simulink model "chap05"  (R2021a)
settings: Solver=FixedStepDiscrete  StartTime=0.0  StopTime=inf  FixedStep=0.001  RelTol=1e-3
undefined symbols (not defined in the file): DiscIntNeverNeededParam, Header, Pose, X, Y, Z
libraries: robotlib x31
(part 5 of 9)

== system chap05/Subsystem16/Subsystem12/Subsystem1 ==
  xx6 : Inport
  xx0 : Inport  Port=2
  xx1 : Inport  Port=3
  xx2 : Inport  Port=4
  vx6 : Inport  Port=5
  vx0 : Inport  Port=6
  vx1 : Inport  Port=7
  vx2 : Inport  Port=8
  Add : Sum
  Add1 : Sum  Inputs=-+
  Add10 : Sum  Inputs=-+
  Add2 : Sum  Inputs=+-
  Add4 : Sum  Inputs=-+
  Add5 : Sum  Inputs=+++
  Add6 : Sum  Inputs=+-
  Add8 : Sum  Inputs=+++
  Add9 : Sum  Inputs=+-
  Constant : Constant  Value=0.75
  Constant1 : Constant  Value=0.85
  Constant3 : Constant  Value=1.2
  Constant{4..5,7..8} (4 alike) : Constant  Value=1.5
  Constant6 : Constant  Value=1.2
  Product{1,3..9} (8 alike) : Product
  utx : Outport
  wires:
  Product7/1 -> Add8/3
  Add6/1 -> Product7/1
  Constant8/1 -> Product7/2
  vx0/1 -> Add6/2
  Product3/1 -> Add5/1
  Add1/1 -> Product3/2
  Constant7/1 -> Product3/1
  xx0/1 -> Add1/1
  vx6/1 -> Add10/2, Add9/1, Add6/1
  vx2/1 -> Add10/1
  vx1/1 -> Add9/2
  xx1/1 -> Add2/2
  xx2/1 -> Add4/1
  Add/1 -> utx/1
  Add5/1 -> Product6/2
  Add2/1 -> Product5/1
  Product1/1 -> Add/2
  Constant1/1 -> Product1/1
  Constant/1 -> Product6/1
  Product6/1 -> Add/1
  Constant3/1 -> Product5/2
  xx6/1 -> Add4/2, Add2/1, Add1/2
  Add4/1 -> Product4/2
  Constant4/1 -> Product4/1
  Product5/1 -> Add5/3
  Product4/1 -> Add5/2
  Add8/1 -> Product1/2
  Constant5/1 -> Product8/1
  Add10/1 -> Product8/2
  Constant6/1 -> Product9/2
  Add9/1 -> Product9/1
  Product8/1 -> Add8/1
  Product9/1 -> Add8/2

== system chap05/Subsystem16/Subsystem12/Subsystem2 ==
  xx6 : Inport
  xx0 : Inport  Port=2
  xx1 : Inport  Port=3
  xx2 : Inport  Port=4
  vx6 : Inport  Port=5
  vx0 : Inport  Port=6
  vx1 : Inport  Port=7
  vx2 : Inport  Port=8
  Add : Sum
  Add1 : Sum  Inputs=-+
  Add10 : Sum  Inputs=-+
  Add2 : Sum  Inputs=+-
  Add4 : Sum  Inputs=-+
  Add5 : Sum  Inputs=+++
  Add6 : Sum  Inputs=+-
  Add8 : Sum  Inputs=+++
  Add9 : Sum  Inputs=+-
  Constant : Constant  Value=0.75
  Constant1 : Constant  Value=0.85
  Constant3 : Constant  Value=1.2
  Constant{4..5,7..8} (4 alike) : Constant  Value=1.5
  Constant6 : Constant  Value=1.2
  Product{1,3..9} (8 alike) : Product
  utx : Outport
  wires:
  Product9/1 -> Add8/2
  Product8/1 -> Add8/1
  Add9/1 -> Product9/1
  Constant6/1 -> Product9/2
  Add10/1 -> Product8/2
  Constant5/1 -> Product8/1
  Add8/1 -> Product1/2
  Product4/1 -> Add5/2
  Product5/1 -> Add5/3
  Constant4/1 -> Product4/1
  Add4/1 -> Product4/2
  xx6/1 -> Add1/2, Add2/1, Add4/2
  Constant3/1 -> Product5/2
  Product6/1 -> Add/1
  Constant/1 -> Product6/1
  Constant1/1 -> Product1/1
  Product1/1 -> Add/2
  Add2/1 -> Product5/1
  Add5/1 -> Product6/2
  Add/1 -> utx/1
  xx2/1 -> Add4/1
  xx1/1 -> Add2/2
  vx1/1 -> Add9/2
  vx2/1 -> Add10/1
  vx6/1 -> Add6/1, Add9/1, Add10/2
  xx0/1 -> Add1/1
  Constant7/1 -> Product3/1
  Add1/1 -> Product3/2
  Product3/1 -> Add5/1
  vx0/1 -> Add6/2
  Constant8/1 -> Product7/2
  Add6/1 -> Product7/1
  Product7/1 -> Add8/3

== system chap05/Subsystem16/Subsystem12/Subsystem3 ==
  xyk : Inport
  xy : Inport  Port=2
  vyk : Inport  Port=3
  vy : Inport  Port=4
  Add : Sum
  Add4 : Sum  Inputs=-+
  Add8 : Sum  Inputs=-+
  Constant : Constant  Value=0.75
  Constant1 : Constant  Value=0.85
  Product1 : Product
  Product6 : Product
  ey : Outport
  wires:
  vyk/1 -> Add8/2
  vy/1 -> Add8/1
  xy/1 -> Add4/1
  Add/1 -> ey/1
  Add4/1 -> Product6/2
  Product1/1 -> Add/2
  Constant1/1 -> Product1/1
  Constant/1 -> Product6/1
  Product6/1 -> Add/1
  xyk/1 -> Add4/2
  Add8/1 -> Product1/2

== system chap05/Subsystem16/Subsystem12/Subsystem4 ==
  xzk : Inport
  xz : Inport  Port=2
  vzk : Inport  Port=3
  vz : Inport  Port=4
  Add : Sum
  Add4 : Sum  Inputs=-+
  Add8 : Sum  Inputs=-+
  Constant : Constant  Value=0.75
  Constant1 : Constant  Value=0.85
  Product1 : Product
  Product6 : Product
  ez : Outport
  wires:
  Add8/1 -> Product1/2
  xzk/1 -> Add4/2
  Product6/1 -> Add/1
  Constant/1 -> Product6/1
  Constant1/1 -> Product1/1
  Product1/1 -> Add/2
  Add4/1 -> Product6/2
  Add/1 -> ez/1
  xz/1 -> Add4/1
  vz/1 -> Add8/1
  vzk/1 -> Add8/2

== system chap05/Subsystem16/Subsystem12/Subsystem5 ==
  xxk : Inport
  xx : Inport  Port=2
  vxk : Inport  Port=3
  vx : Inport  Port=4
  Add : Sum
  Add4 : Sum  Inputs=-+
  Add8 : Sum  Inputs=-+
  Constant : Constant  Value=0.75
  Constant1 : Constant  Value=0.85
  Product1 : Product
  Product6 : Product
  ex : Outport
  wires:
  Add8/1 -> Product1/2
  xxk/1 -> Add4/2
  Product6/1 -> Add/1
  Constant/1 -> Product6/1
  Constant1/1 -> Product1/1
  Product1/1 -> Add/2
  Add4/1 -> Product6/2
  Add/1 -> ex/1
  xx/1 -> Add4/1
  vx/1 -> Add8/1
  vxk/1 -> Add8/2

== system chap05/Subsystem16/Subsystem12/Subsystem6 ==
  xx6 : Inport
  xx0 : Inport  Port=2
  xx1 : Inport  Port=3
  xx2 : Inport  Port=4
  vx6 : Inport  Port=5
  vx0 : Inport  Port=6
  vx1 : Inport  Port=7
  vx2 : Inport  Port=8
  Add : Sum
  Add1 : Sum  Inputs=-+
  Add10 : Sum  Inputs=-+
  Add2 : Sum  Inputs=+-
  Add4 : Sum  Inputs=-+
  Add5 : Sum  Inputs=+++
  Add6 : Sum  Inputs=+-
  Add8 : Sum  Inputs=+++
  Add9 : Sum  Inputs=+-
  Constant : Constant  Value=0.75
  Constant1 : Constant  Value=0.85
  Constant3 : Constant  Value=1.2
  Constant{4..5,7..8} (4 alike) : Constant  Value=1.5
  Constant6 : Constant  Value=1.2
  Product{1,3..9} (8 alike) : Product
  utx : Outport
  wires:
  Product9/1 -> Add8/2
  Product8/1 -> Add8/1
  Add9/1 -> Product9/1
  Constant6/1 -> Product9/2
  Add10/1 -> Product8/2
  Constant5/1 -> Product8/1
  Add8/1 -> Product1/2
  Product4/1 -> Add5/2
  Product5/1 -> Add5/3
  Constant4/1 -> Product4/1
  Add4/1 -> Product4/2
  xx6/1 -> Add1/2, Add2/1, Add4/2
  Constant3/1 -> Product5/2
  Product6/1 -> Add/1
  Constant/1 -> Product6/1
  Constant1/1 -> Product1/1
  Product1/1 -> Add/2
  Add2/1 -> Product5/1
  Add5/1 -> Product6/2
  Add/1 -> utx/1
  xx2/1 -> Add4/1
  xx1/1 -> Add2/2
  vx1/1 -> Add9/2
  vx2/1 -> Add10/1
  vx6/1 -> Add6/1, Add9/1, Add10/2
  xx0/1 -> Add1/1
  Constant7/1 -> Product3/1
  Add1/1 -> Product3/2
  Product3/1 -> Add5/1
  vx0/1 -> Add6/2
  Constant8/1 -> Product7/2
  Add6/1 -> Product7/1
  Product7/1 -> Add8/3

== system chap05/Subsystem16/Subsystem14/L+B ==
  Add : Sum
  Constant1 : Constant  Value=|
      | [2.5 0 0 0 0 0
      |      0 2.8 0 0 0 0
      |      0 0 2.8 0 0 0
      |      0 0 0 2.5 0 0
      |      0 0 0 0 2.7 0
      |      0 0 0 0 0 2.7]
  Constant2 : Constant  Value=|
      | [0.0 0.8 0.5 0.0 0.0 1.2
      |      0.8 0.0 0.0 0.5 0.0 1.5
      |      0.5 0.0 0.0 0.8 1.5 0.0
      |      0.0 0.5 0.8 0.0 1.2 0.0
      |      0.0 0.0 1.5 1.2 0.0 0.0
      |      1.2 1.5 0.0 0.0 0.0 0.0]
  Constant3 : Constant  Value=|
      | [0.0 0.0 0.0 0.0 0.0 0.0
      |      0.0 0.0 0.0 0.0 0.0 0.0
      |      0.0 0.0 0.0 0.0 0.0 0.0
      |      0.0 0.0 0.0 0.0 0.0 0.0
      |      0.0 0.0 0.0 0.0 1.5 0.0
      |      0.0 0.0 0.0 0.0 0.0 1.5]
  Subtract : Sum  Inputs=+-
  u : Outport
  wires:
  Constant2/1 -> Subtract/2
  Constant1/1 -> Subtract/1
  Subtract/1 -> Add/1
  Add/1 -> u/1
  Constant3/1 -> Add/2

== system chap05/Subsystem16/Subsystem14/Subsystem1 ==
  xy1 : Inport
  xy2 : Inport  Port=2
  xy3 : Inport  Port=3
  xy6 : Inport  Port=4
  vy1 : Inport  Port=5
  vy2 : Inport  Port=6
  vy3 : Inport  Port=7
  vy6 : Inport  Port=8
  Add : Sum
  Add{1,4,6,8} (4 alike) : Sum  Inputs=-+
  Add2 : Sum  Inputs=+-
  Add5 : Sum  Inputs=+++
  Add7 : Sum  Inputs=+-
  Add9 : Sum  Inputs=+++
  Constant : Constant  Value=0.75
  Constant1 : Constant  Value=0.85
  Constant3 : Constant  Value=0.5
  Constant4 : Constant  Value=0.8
  Constant5 : Constant  Value=1.2
  Constant7 : Constant  Value=0.5
  Constant8 : Constant  Value=0.8
  Constant9 : Constant  Value=1.2
  Product{1,3..9} (8 alike) : Product
  p2y : Outport
  wires:
  Add9/1 -> Product1/2
  Product4/1 -> Add5/2
  Product5/1 -> Add5/3
  Constant3/1 -> Product4/1
  Add4/1 -> Product4/2
  xy1/1 -> Add1/2, Add4/2, Add2/1
  Constant4/1 -> Product5/2
  Product6/1 -> Add/1
  Constant/1 -> Product6/1
  Constant1/1 -> Product1/1
  Product1/1 -> Add/2
  Add2/1 -> Product5/1
  Add5/1 -> Product6/2
  Add/1 -> p2y/1
  xy3/1 -> Add4/1
  xy2/1 -> Add2/2
  xy6/1 -> Add1/1
  Constant5/1 -> Product3/1
  Add1/1 -> Product3/2
  Product3/1 -> Add5/1
  Product7/1 -> Add9/1
  Add6/1 -> Product7/2
  Constant9/1 -> Product7/1
  vy6/1 -> Add6/1
  vy2/1 -> Add7/2
  vy3/1 -> Add8/1
  Add7/1 -> Product9/1
  Constant8/1 -> Product9/2
  vy1/1 -> Add7/1, Add8/2, Add6/2
  Add8/1 -> Product8/2
  Constant7/1 -> Product8/1
  Product9/1 -> Add9/3
  Product8/1 -> Add9/2

== system chap05/Subsystem16/Subsystem14/Subsystem2 ==
  xz1 : Inport
  xx2 : Inport  Port=2
  xz3 : Inport  Port=3
  xz6 : Inport  Port=4
  vz1 : Inport  Port=5
  vz2 : Inport  Port=6
  vz3 : Inport  Port=7
  vz6 : Inport  Port=8
  Add : Sum
  Add{1,4,6,8} (4 alike) : Sum  Inputs=-+
  Add2 : Sum  Inputs=+-
  Add5 : Sum  Inputs=+++
  Add7 : Sum  Inputs=+-
  Add9 : Sum  Inputs=+++
  Constant : Constant  Value=0.75
  Constant1 : Constant  Value=0.85
  Constant3 : Constant  Value=0.5
  Constant4 : Constant  Value=0.8
  Constant5 : Constant  Value=1.2
  Constant7 : Constant  Value=0.5
  Constant8 : Constant  Value=0.8
  Constant9 : Constant  Value=1.2
  Product{1,3..9} (8 alike) : Product
  p3z : Outport
  wires:
  Product8/1 -> Add9/2
  Product9/1 -> Add9/3
  Constant7/1 -> Product8/1
  Add8/1 -> Product8/2
  vz1/1 -> Add6/2, Add8/2, Add7/1
  Constant8/1 -> Product9/2
  Add7/1 -> Product9/1
  vz3/1 -> Add8/1
  vz2/1 -> Add7/2
  vz6/1 -> Add6/1
  Constant9/1 -> Product7/1
  Add6/1 -> Product7/2
  Product7/1 -> Add9/1
  Product3/1 -> Add5/1
  Add1/1 -> Product3/2
  Constant5/1 -> Product3/1
  xz6/1 -> Add1/1
  xx2/1 -> Add2/2
  xz3/1 -> Add4/1
  Add/1 -> p3z/1
  Add5/1 -> Product6/2
  Add2/1 -> Product5/1
  Product1/1 -> Add/2
  Constant1/1 -> Product1/1
  Constant/1 -> Product6/1
  Product6/1 -> Add/1
  Constant4/1 -> Product5/2
  xz1/1 -> Add2/1, Add4/2, Add1/2
  Add4/1 -> Product4/2
  Constant3/1 -> Product4/1
  Product5/1 -> Add5/3
  Product4/1 -> Add5/2
  Add9/1 -> Product1/2

== system chap05/Subsystem16/Subsystem14/Subsystem3 ==
  xyk : Inport
  xy : Inport  Port=2
  vyk : Inport  Port=3
  vy : Inport  Port=4
  Add : Sum
  Add4 : Sum  Inputs=-+
  Add8 : Sum  Inputs=-+
  Constant : Constant  Value=0.75
  Constant1 : Constant  Value=0.85
  Product1 : Product
  Product6 : Product
  ey : Outport
  wires:
  vyk/1 -> Add8/2
  vy/1 -> Add8/1
  xy/1 -> Add4/1
  Add/1 -> ey/1
  Add4/1 -> Product6/2
  Product1/1 -> Add/2
  Constant1/1 -> Product1/1
  Constant/1 -> Product6/1
  Product6/1 -> Add/1
  xyk/1 -> Add4/2
  Add8/1 -> Product1/2

== system chap05/Subsystem16/Subsystem14/Subsystem4 ==
  xzk : Inport
  xz : Inport  Port=2
  vzk : Inport  Port=3
  vz : Inport  Port=4
  Add : Sum
  Add4 : Sum  Inputs=-+
  Add8 : Sum  Inputs=-+
  Constant : Constant  Value=0.75
  Constant1 : Constant  Value=0.85
  Product1 : Product
  Product6 : Product
  ez : Outport
  wires:
  Add8/1 -> Product1/2
  xzk/1 -> Add4/2
  Product6/1 -> Add/1
  Constant/1 -> Product6/1
  Constant1/1 -> Product1/1
  Product1/1 -> Add/2
  Add4/1 -> Product6/2
  Add/1 -> ez/1
  xz/1 -> Add4/1
  vz/1 -> Add8/1
  vzk/1 -> Add8/2

== system chap05/Subsystem16/Subsystem14/Subsystem5 ==
  xxk : Inport
  xx : Inport  Port=2
  vxk : Inport  Port=3
  vx : Inport  Port=4
  Add : Sum
  Add4 : Sum  Inputs=-+
  Add8 : Sum  Inputs=-+
  Constant : Constant  Value=0.75
  Constant1 : Constant  Value=0.85
  Product1 : Product
  Product6 : Product
  ex : Outport
  wires:
  Add8/1 -> Product1/2
  xxk/1 -> Add4/2
  Product6/1 -> Add/1
  Constant/1 -> Product6/1
  Constant1/1 -> Product1/1
  Product1/1 -> Add/2
  Add4/1 -> Product6/2
  Add/1 -> ex/1
  xx/1 -> Add4/1
  vx/1 -> Add8/1
  vxk/1 -> Add8/2

== system chap05/Subsystem16/Subsystem14/Subsystem6 ==
  xx1 : Inport
  xx2 : Inport  Port=2
  xx3 : Inport  Port=3
  xx6 : Inport  Port=4
  vx1 : Inport  Port=5
  vx2 : Inport  Port=6
  vx3 : Inport  Port=7
  vx6 : Inport  Port=8
  Add : Sum
  Add{1,4,6,8} (4 alike) : Sum  Inputs=-+
  Add2 : Sum  Inputs=+-
  Add5 : Sum  Inputs=+++
  Add7 : Sum  Inputs=+-
  Add9 : Sum  Inputs=+++
  Constant : Constant  Value=0.75
  Constant1 : Constant  Value=0.85
  Constant3 : Constant  Value=0.5
  Constant4 : Constant  Value=0.8
  Constant5 : Constant  Value=1.2
  Constant7 : Constant  Value=0.5
  Constant8 : Constant  Value=0.8
  Constant9 : Constant  Value=1.2
  Product{1,3..9} (8 alike) : Product
  p1x : Outport
  wires:
  Product8/1 -> Add9/2
  Product9/1 -> Add9/3
  Constant7/1 -> Product8/1
  Add8/1 -> Product8/2
  vx1/1 -> Add6/2, Add8/2, Add7/1
  Constant8/1 -> Product9/2
  Add7/1 -> Product9/1
  vx3/1 -> Add8/1
  vx2/1 -> Add7/2
  vx6/1 -> Add6/1
  Constant9/1 -> Product7/1
  Add6/1 -> Product7/2
  Product7/1 -> Add9/1
  Product3/1 -> Add5/1
  Add1/1 -> Product3/2
  Constant5/1 -> Product3/1
  xx6/1 -> Add1/1
  xx2/1 -> Add2/2
  xx3/1 -> Add4/1
  Add/1 -> p1x/1
  Add5/1 -> Product6/2
  Add2/1 -> Product5/1
  Product1/1 -> Add/2
  Constant1/1 -> Product1/1
  Constant/1 -> Product6/1
  Product6/1 -> Add/1
  Constant4/1 -> Product5/2
  xx1/1 -> Add2/1, Add4/2, Add1/2
  Add4/1 -> Product4/2
  Constant3/1 -> Product4/1
  Product5/1 -> Add5/3
  Product4/1 -> Add5/2
  Add9/1 -> Product1/2

== system chap05/Subsystem16/Subsystem15/L+B ==
  Add : Sum
  Constant1 : Constant  Value=|
      | [2.5 0 0 0 0 0
      |      0 2.8 0 0 0 0
      |      0 0 2.8 0 0 0
      |      0 0 0 2.5 0 0
      |      0 0 0 0 2.7 0
      |      0 0 0 0 0 2.7]
  Constant2 : Constant  Value=|
      | [0.0 0.8 0.5 0.0 0.0 1.2
      |      0.8 0.0 0.0 0.5 0.0 1.5
      |      0.5 0.0 0.0 0.8 1.5 0.0
      |      0.0 0.5 0.8 0.0 1.2 0.0
      |      0.0 0.0 1.5 1.2 0.0 0.0
      |      1.2 1.5 0.0 0.0 0.0 0.0]
  Constant3 : Constant  Value=|
      | [0.0 0.0 0.0 0.0 0.0 0.0
      |      0.0 0.0 0.0 0.0 0.0 0.0
      |      0.0 0.0 0.0 0.0 0.0 0.0
      |      0.0 0.0 0.0 0.0 0.0 0.0
      |      0.0 0.0 0.0 0.0 1.5 0.0
      |      0.0 0.0 0.0 0.0 0.0 1.5]
  Subtract : Sum  Inputs=+-
  u : Outport
  wires:
  Constant2/1 -> Subtract/2
  Constant1/1 -> Subtract/1
  Subtract/1 -> Add/1
  Add/1 -> u/1
  Constant3/1 -> Add/2

== system chap05/Subsystem16/Subsystem15/Subsystem1 ==
  xy2 : Inport
  xy1 : Inport  Port=2
  xy4 : Inport  Port=3
  xy6 : Inport  Port=4
  vy2 : Inport  Port=5
  vy1 : Inport  Port=6
  vy4 : Inport  Port=7
  vy6 : Inport  Port=8
  Add : Sum
  Add{1,4,6,8} (4 alike) : Sum  Inputs=-+
  Add2 : Sum  Inputs=+-
  Add5 : Sum  Inputs=+++
  Add7 : Sum  Inputs=+-
  Add9 : Sum  Inputs=+++
  Constant : Constant  Value=0.75
  Constant1 : Constant  Value=0.85
  Constant2 : Constant  Value=0.5
  Constant3 : Constant  Value=0.5
  Constant4 : Constant  Value=0.8
  Constant5 : Constant  Value=1.5
  Constant6 : Constant  Value=0.8
  Constant7 : Constant  Value=1.5
  Product{1,3..9} (8 alike) : Product
  p2y : Outport
  wires:
  Product8/1 -> Add9/2
  Product9/1 -> Add9/3
  Constant2/1 -> Product8/1
  Add8/1 -> Product8/2
  vy2/1 -> Add6/2, Add8/2, Add7/1
  Constant6/1 -> Product9/2
  Add7/1 -> Product9/1
  vy4/1 -> Add8/1
  vy1/1 -> Add7/2
  vy6/1 -> Add6/1
  Constant7/1 -> Product7/1
  Add6/1 -> Product7/2
  Product7/1 -> Add9/1
  Product3/1 -> Add5/1
  Add1/1 -> Product3/2
  Constant5/1 -> Product3/1
  xy6/1 -> Add1/1
  xy1/1 -> Add2/2
  xy4/1 -> Add4/1
  Add5/1 -> Product6/2
  Add2/1 -> Product5/1
  Product1/1 -> Add/2
  Constant1/1 -> Product1/1
  Constant/1 -> Product6/1
  Product6/1 -> Add/1
  Constant4/1 -> Product5/2
  xy2/1 -> Add2/1, Add4/2, Add1/2
  Add4/1 -> Product4/2
  Constant3/1 -> Product4/1
  Product5/1 -> Add5/3
  Product4/1 -> Add5/2
  Add9/1 -> Product1/2
  Add/1 -> p2y/1

== system chap05/Subsystem16/Subsystem15/Subsystem2 ==
  xz2 : Inport
  xz1 : Inport  Port=2
  xz4 : Inport  Port=3
  xz6 : Inport  Port=4
  vz2 : Inport  Port=5
  vz1 : Inport  Port=6
  vz4 : Inport  Port=7
  vz6 : Inport  Port=8
  Add : Sum
  Add{1,4,6,8} (4 alike) : Sum  Inputs=-+
  Add2 : Sum  Inputs=+-
  Add5 : Sum  Inputs=+++
  Add7 : Sum  Inputs=+-
  Add9 : Sum  Inputs=+++
  Constant : Constant  Value=0.75
  Constant1 : Constant  Value=0.85
  Constant2 : Constant  Value=0.5
  Constant3 : Constant  Value=0.5
  Constant4 : Constant  Value=0.8
  Constant5 : Constant  Value=1.5
  Constant6 : Constant  Value=0.8
  Constant7 : Constant  Value=1.5
  Product{1,3..9} (8 alike) : Product
  p2z : Outport
  wires:
  Add9/1 -> Product1/2
  Product4/1 -> Add5/2
  Product5/1 -> Add5/3
  Constant3/1 -> Product4/1
  Add4/1 -> Product4/2
  xz2/1 -> Add1/2, Add4/2, Add2/1
  Constant4/1 -> Product5/2
  Product6/1 -> Add/1
  Constant/1 -> Product6/1
  Constant1/1 -> Product1/1
  Product1/1 -> Add/2
  Add2/1 -> Product5/1
  Add5/1 -> Product6/2
  Add/1 -> p2z/1
  xz4/1 -> Add4/1
  xz1/1 -> Add2/2
  xz6/1 -> Add1/1
  Constant5/1 -> Product3/1
  Add1/1 -> Product3/2
  Product3/1 -> Add5/1
  Product7/1 -> Add9/1
  Add6/1 -> Product7/2
  Constant7/1 -> Product7/1
  vz6/1 -> Add6/1
  vz1/1 -> Add7/2
  vz4/1 -> Add8/1
  Add7/1 -> Product9/1
  Constant6/1 -> Product9/2
  vz2/1 -> Add7/1, Add8/2, Add6/2
  Add8/1 -> Product8/2
  Constant2/1 -> Product8/1
  Product9/1 -> Add9/3
  Product8/1 -> Add9/2

== system chap05/Subsystem16/Subsystem15/Subsystem3 ==
  xyk : Inport
  xy : Inport  Port=2
  vyk : Inport  Port=3
  vy : Inport  Port=4
  Add : Sum
  Add4 : Sum  Inputs=-+
  Add8 : Sum  Inputs=-+
  Constant : Constant  Value=0.75
  Constant1 : Constant  Value=0.85
  Product1 : Product
  Product6 : Product
  ey : Outport
  wires:
  vyk/1 -> Add8/2
  vy/1 -> Add8/1
  xy/1 -> Add4/1
  Add/1 -> ey/1
  Add4/1 -> Product6/2
  Product1/1 -> Add/2
  Constant1/1 -> Product1/1
  Constant/1 -> Product6/1
  Product6/1 -> Add/1
  xyk/1 -> Add4/2
  Add8/1 -> Product1/2

== system chap05/Subsystem16/Subsystem15/Subsystem4 ==
  xzk : Inport
  xz : Inport  Port=2
  vzk : Inport  Port=3
  vz : Inport  Port=4
  Add : Sum
  Add4 : Sum  Inputs=-+
  Add8 : Sum  Inputs=-+
  Constant : Constant  Value=0.75
  Constant1 : Constant  Value=0.85
  Product1 : Product
  Product6 : Product
  ez : Outport
  wires:
  Add8/1 -> Product1/2
  xzk/1 -> Add4/2
  Product6/1 -> Add/1
  Constant/1 -> Product6/1
  Constant1/1 -> Product1/1
  Product1/1 -> Add/2
  Add4/1 -> Product6/2
  Add/1 -> ez/1
  xz/1 -> Add4/1
  vz/1 -> Add8/1
  vzk/1 -> Add8/2

== system chap05/Subsystem16/Subsystem15/Subsystem5 ==
  xxk : Inport
  xx : Inport  Port=2
  vxk : Inport  Port=3
  vx : Inport  Port=4
  Add : Sum
  Add4 : Sum  Inputs=-+
  Add8 : Sum  Inputs=-+
  Constant : Constant  Value=0.75
  Constant1 : Constant  Value=0.85
  Product1 : Product
  Product6 : Product
  ex : Outport
  wires:
  Add8/1 -> Product1/2
  xxk/1 -> Add4/2
  Product6/1 -> Add/1
  Constant/1 -> Product6/1
  Constant1/1 -> Product1/1
  Product1/1 -> Add/2
  Add4/1 -> Product6/2
  Add/1 -> ex/1
  xx/1 -> Add4/1
  vx/1 -> Add8/1
  vxk/1 -> Add8/2

== system chap05/Subsystem16/Subsystem15/Subsystem6 ==
  xx2 : Inport
  xx1 : Inport  Port=2
  xx4 : Inport  Port=3
  xx6 : Inport  Port=4
  vx2 : Inport  Port=5
  vx1 : Inport  Port=6
  vx4 : Inport  Port=7
  vx6 : Inport  Port=8
  Add : Sum
  Add{1,4,6,8} (4 alike) : Sum  Inputs=-+
  Add2 : Sum  Inputs=+-
  Add5 : Sum  Inputs=+++
  Add7 : Sum  Inputs=+-
  Add9 : Sum  Inputs=+++
  Constant : Constant  Value=0.75
  Constant1 : Constant  Value=0.85
  Constant2 : Constant  Value=0.5
  Constant3 : Constant  Value=0.5
  Constant4 : Constant  Value=0.8
  Constant5 : Constant  Value=1.5
  Constant6 : Constant  Value=0.8
  Constant7 : Constant  Value=1.5
  Product{1,3..9} (8 alike) : Product
  p2x : Outport
  wires:
  Add9/1 -> Product1/2
  Product4/1 -> Add5/2
  Product5/1 -> Add5/3
  Constant3/1 -> Product4/1
  Add4/1 -> Product4/2
  xx2/1 -> Add1/2, Add4/2, Add2/1
  Constant4/1 -> Product5/2
  Product6/1 -> Add/1
  Constant/1 -> Product6/1
  Constant1/1 -> Product1/1
  Product1/1 -> Add/2
  Add2/1 -> Product5/1
  Add5/1 -> Product6/2
  xx4/1 -> Add4/1
  xx1/1 -> Add2/2
  xx6/1 -> Add1/1
  Constant5/1 -> Product3/1
  Add1/1 -> Product3/2
  Product3/1 -> Add5/1
  Product7/1 -> Add9/1
  Add6/1 -> Product7/2
  Constant7/1 -> Product7/1
  vx6/1 -> Add6/1
  vx1/1 -> Add7/2
  vx4/1 -> Add8/1
  Add7/1 -> Product9/1
  Constant6/1 -> Product9/2
  vx2/1 -> Add7/1, Add8/2, Add6/2
  Add8/1 -> Product8/2
  Constant2/1 -> Product8/1
  Product9/1 -> Add9/3
  Product8/1 -> Add9/2
  Add/1 -> p2x/1

== system chap05/Subsystem16/Subsystem16/L+B ==
  Add : Sum
  Constant1 : Constant  Value=|
      | [2.5 0 0 0 0 0
      |      0 2.8 0 0 0 0
      |      0 0 2.8 0 0 0
      |      0 0 0 2.5 0 0
      |      0 0 0 0 2.7 0
      |      0 0 0 0 0 2.7]
  Constant2 : Constant  Value=|
      | [0.0 0.8 0.5 0.0 0.0 1.2
      |      0.8 0.0 0.0 0.5 0.0 1.5
      |      0.5 0.0 0.0 0.8 1.5 0.0
      |      0.0 0.5 0.8 0.0 1.2 0.0
      |      0.0 0.0 1.5 1.2 0.0 0.0
      |      1.2 1.5 0.0 0.0 0.0 0.0]
  Constant3 : Constant  Value=|
      | [0.0 0.0 0.0 0.0 0.0 0.0
      |      0.0 0.0 0.0 0.0 0.0 0.0
      |      0.0 0.0 0.0 0.0 0.0 0.0
      |      0.0 0.0 0.0 0.0 0.0 0.0
      |      0.0 0.0 0.0 0.0 1.5 0.0
      |      0.0 0.0 0.0 0.0 0.0 1.5]
  Subtract : Sum  Inputs=+-
  u : Outport
  wires:
  Constant2/1 -> Subtract/2
  Constant1/1 -> Subtract/1
  Subtract/1 -> Add/1
  Add/1 -> u/1
  Constant3/1 -> Add/2

== system chap05/Subsystem16/Subsystem16/Subsystem1 ==
  xxk : Inport
  xx : Inport  Port=2
  vxk : Inport  Port=3
  vx : Inport  Port=4
  Add : Sum
  Add4 : Sum  Inputs=-+
  Add8 : Sum  Inputs=-+
  Constant : Constant  Value=0.75
  Constant1 : Constant  Value=0.85
  Product1 : Product
  Product6 : Product
  ex : Outport
  wires:
  vxk/1 -> Add8/2
  vx/1 -> Add8/1
  xx/1 -> Add4/1
  Add/1 -> ex/1
  Add4/1 -> Product6/2
  Product1/1 -> Add/2
  Constant1/1 -> Product1/1
  Constant/1 -> Product6/1
  Product6/1 -> Add/1
  xxk/1 -> Add4/2
  Add8/1 -> Product1/2

== system chap05/Subsystem16/Subsystem16/Subsystem2 ==
  xy5 : Inport
  xy0 : Inport  Port=2
  xy3 : Inport  Port=3
  xy4 : Inport  Port=4
  vy5 : Inport  Port=5
  vy0 : Inport  Port=6
  vy3 : Inport  Port=7
  vy4 : Inport  Port=8
  Add : Sum
  Add1 : Sum  Inputs=-+
  Add10 : Sum  Inputs=-+
  Add2 : Sum  Inputs=+-
  Add4 : Sum  Inputs=-+
  Add5 : Sum  Inputs=+++
  Add6 : Sum  Inputs=+-
  Add8 : Sum  Inputs=+++
  Add9 : Sum  Inputs=+-
  Constant : Constant  Value=0.75
  Constant1 : Constant  Value=0.85
  Constant3 : Constant  Value=1.2
  Constant{4,6..8} (4 alike) : Constant  Value=1.5
  Constant5 : Constant  Value=1.2
  Product{1,3..9} (8 alike) : Product
  uty : Outport
  wires:
  vy0/1 -> Add6/2
  Constant8/1 -> Product7/2
  Add6/1 -> Product7/1
  Product7/1 -> Add8/3
  Product3/1 -> Add5/1
  xy0/1 -> Add1/1
  Add1/1 -> Product3/2
  Constant7/1 -> Product3/1
  Product9/1 -> Add8/2
  Product8/1 -> Add8/1
  Add9/1 -> Product9/1
  Constant6/1 -> Product9/2
  Add10/1 -> Product8/2
  Constant5/1 -> Product8/1
  Add8/1 -> Product1/2
  Product4/1 -> Add5/2
  Product5/1 -> Add5/3
  Constant3/1 -> Product4/1
  Add4/1 -> Product4/2
  xy5/1 -> Add2/1, Add4/2, Add1/2
  Constant4/1 -> Product5/2
  Product6/1 -> Add/1
  Constant/1 -> Product6/1
  Constant1/1 -> Product1/1
  Product1/1 -> Add/2
  Add2/1 -> Product5/1
  Add5/1 -> Product6/2
  Add/1 -> uty/1
  xy4/1 -> Add4/1
  xy3/1 -> Add2/2
  vy3/1 -> Add9/2
  vy4/1 -> Add10/1
  vy5/1 -> Add9/1, Add6/1, Add10/2

== system chap05/Subsystem16/Subsystem16/Subsystem3 ==
  xyk : Inport
  xy : Inport  Port=2
  vyk : Inport  Port=3
  vy : Inport  Port=4
  Add : Sum
  Add4 : Sum  Inputs=-+
  Add8 : Sum  Inputs=-+
  Constant : Constant  Value=0.75
  Constant1 : Constant  Value=0.85
  Product1 : Product
  Product6 : Product
  ey : Outport
  wires:
  Add8/1 -> Product1/2
  xyk/1 -> Add4/2
  Product6/1 -> Add/1
  Constant/1 -> Product6/1
  Constant1/1 -> Product1/1
  Product1/1 -> Add/2
  Add4/1 -> Product6/2
  Add/1 -> ey/1
  xy/1 -> Add4/1
  vy/1 -> Add8/1
  vyk/1 -> Add8/2

== system chap05/Subsystem16/Subsystem16/Subsystem4 ==
  xzk : Inport
  xz : Inport  Port=2
  vzk : Inport  Port=3
  vz : Inport  Port=4
  Add : Sum
  Add4 : Sum  Inputs=-+
  Add8 : Sum  Inputs=-+
  Constant : Constant  Value=0.75
  Constant1 : Constant  Value=0.85
  Product1 : Product
  Product6 : Product
  ez : Outport
  wires:
  vzk/1 -> Add8/2
  vz/1 -> Add8/1
  xz/1 -> Add4/1
  Add/1 -> ez/1
  Add4/1 -> Product6/2
  Product1/1 -> Add/2
  Constant1/1 -> Product1/1
  Constant/1 -> Product6/1
  Product6/1 -> Add/1
  xzk/1 -> Add4/2
  Add8/1 -> Product1/2

== system chap05/Subsystem16/Subsystem16/Subsystem5 ==
  xz5 : Inport
  xz0 : Inport  Port=2
  xz3 : Inport  Port=3
  xz4 : Inport  Port=4
  vz5 : Inport  Port=5
  vz0 : Inport  Port=6
  vz3 : Inport  Port=7
  vz4 : Inport  Port=8
  Add : Sum
  Add1 : Sum  Inputs=-+
  Add10 : Sum  Inputs=-+
  Add2 : Sum  Inputs=+-
  Add4 : Sum  Inputs=-+
  Add5 : Sum  Inputs=+++
  Add6 : Sum  Inputs=+-
  Add8 : Sum  Inputs=+++
  Add9 : Sum  Inputs=+-
  Constant : Constant  Value=0.75
  Constant1 : Constant  Value=0.85
  Constant3 : Constant  Value=1.2
  Constant{4,6..8} (4 alike) : Constant  Value=1.5
  Constant5 : Constant  Value=1.2
  Product{1,3..9} (8 alike) : Product
  utz : Outport
  wires:
  vz5/1 -> Add10/2, Add6/1, Add9/1
  vz4/1 -> Add10/1
  vz3/1 -> Add9/2
  xz3/1 -> Add2/2
  xz4/1 -> Add4/1
  Add/1 -> utz/1
  Add5/1 -> Product6/2
  Add2/1 -> Product5/1
  Product1/1 -> Add/2
  Constant1/1 -> Product1/1
  Constant/1 -> Product6/1
  Product6/1 -> Add/1
  Constant4/1 -> Product5/2
  xz5/1 -> Add1/2, Add4/2, Add2/1
  Add4/1 -> Product4/2
  Constant3/1 -> Product4/1
  Product5/1 -> Add5/3
  Product4/1 -> Add5/2
  Add8/1 -> Product1/2
  Constant5/1 -> Product8/1
  Add10/1 -> Product8/2
  Constant6/1 -> Product9/2
  Add9/1 -> Product9/1
  Product8/1 -> Add8/1
  Product9/1 -> Add8/2
  Constant7/1 -> Product3/1
  Add1/1 -> Product3/2
  xz0/1 -> Add1/1
  Product3/1 -> Add5/1
  Product7/1 -> Add8/3
  Add6/1 -> Product7/1
  Constant8/1 -> Product7/2
  vz0/1 -> Add6/2

== system chap05/Subsystem16/Subsystem16/Subsystem6 ==
  xx5 : Inport
  xx0 : Inport  Port=2
  xx3 : Inport  Port=3
  xx4 : Inport  Port=4
  vx5 : Inport  Port=5
  vx0 : Inport  Port=6
  vx3 : Inport  Port=7
  vx4 : Inport  Port=8
  Add : Sum
  Add1 : Sum  Inputs=-+
  Add10 : Sum  Inputs=-+
  Add2 : Sum  Inputs=+-
  Add4 : Sum  Inputs=-+
  Add5 : Sum  Inputs=+++
  Add6 : Sum  Inputs=+-
  Add8 : Sum  Inputs=+++
  Add9 : Sum  Inputs=+-
  Constant : Constant  Value=0.75
  Constant1 : Constant  Value=0.85
  Constant3 : Constant  Value=1.2
  Constant{4,6..8} (4 alike) : Constant  Value=1.5
  Constant5 : Constant  Value=1.2
  Product{1,3..9} (8 alike) : Product
  utx : Outport
  wires:
  vx5/1 -> Add10/2, Add6/1, Add9/1
  vx4/1 -> Add10/1
  vx3/1 -> Add9/2
  xx3/1 -> Add2/2
  xx4/1 -> Add4/1
  Add/1 -> utx/1
  Add5/1 -> Product6/2
  Add2/1 -> Product5/1
  Product1/1 -> Add/2
  Constant1/1 -> Product1/1
  Constant/1 -> Product6/1
  Product6/1 -> Add/1
  Constant4/1 -> Product5/2
  xx5/1 -> Add1/2, Add4/2, Add2/1
  Add4/1 -> Product4/2
  Constant3/1 -> Product4/1
  Product5/1 -> Add5/3
  Product4/1 -> Add5/2
  Add8/1 -> Product1/2
  Constant5/1 -> Product8/1
  Add10/1 -> Product8/2
  Constant6/1 -> Product9/2
  Add9/1 -> Product9/1
  Product8/1 -> Add8/1
  Product9/1 -> Add8/2
  Constant7/1 -> Product3/1
  Add1/1 -> Product3/2
  xx0/1 -> Add1/1
  Product3/1 -> Add5/1
  Product7/1 -> Add8/3
  Add6/1 -> Product7/1
  Constant8/1 -> Product7/2
  vx0/1 -> Add6/2

== system chap05/Subsystem16/Subsystem17/L+B ==
  Add : Sum
  Constant1 : Constant  Value=|
      | [2.5 0 0 0 0 0
      |      0 2.8 0 0 0 0
      |      0 0 2.8 0 0 0
      |      0 0 0 2.5 0 0
      |      0 0 0 0 2.7 0
      |      0 0 0 0 0 2.7]
  Constant2 : Constant  Value=|
      | [0.0 0.8 0.5 0.0 0.0 1.2
      |      0.8 0.0 0.0 0.5 0.0 1.5
      |      0.5 0.0 0.0 0.8 1.5 0.0
      |      0.0 0.5 0.8 0.0 1.2 0.0
      |      0.0 0.0 1.5 1.2 0.0 0.0
      |      1.2 1.5 0.0 0.0 0.0 0.0]
  Constant3 : Constant  Value=|
      | [0.0 0.0 0.0 0.0 0.0 0.0
      |      0.0 0.0 0.0 0.0 0.0 0.0
      |      0.0 0.0 0.0 0.0 0.0 0.0
      |      0.0 0.0 0.0 0.0 0.0 0.0
      |      0.0 0.0 0.0 0.0 1.5 0.0
      |      0.0 0.0 0.0 0.0 0.0 1.5]
  Subtract : Sum  Inputs=+-
  u : Outport
  wires:
  Constant2/1 -> Subtract/2
  Constant1/1 -> Subtract/1
  Subtract/1 -> Add/1
  Add/1 -> u/1
  Constant3/1 -> Add/2

== system chap05/Subsystem16/Subsystem17/Subsystem1 ==
  xy3 : Inport
  xy1 : Inport  Port=2
  xy4 : Inport  Port=3
  xy5 : Inport  Port=4
  vy3 : Inport  Port=5
  vy1 : Inport  Port=6
  vy4 : Inport  Port=7
  vy5 : Inport  Port=8
  Add : Sum
  Add{1,4,6,8} (4 alike) : Sum  Inputs=-+
  Add2 : Sum  Inputs=+-
  Add5 : Sum  Inputs=+++
  Add7 : Sum  Inputs=+-
  Add9 : Sum  Inputs=+++
  Constant : Constant  Value=0.75
  Constant1 : Constant  Value=0.85
  Constant2 : Constant  Value=0.8
  Constant3 : Constant  Value=0.8
  Constant4 : Constant  Value=0.5
  Constant5 : Constant  Value=1.5
  Constant6 : Constant  Value=0.5
  Constant7 : Constant  Value=1.5
  Product{1,3..9} (8 alike) : Product
  p3y : Outport
  wires:
  Add9/1 -> Product1/2
  Product4/1 -> Add5/2
  Product5/1 -> Add5/3
  Constant3/1 -> Product4/1
  Add4/1 -> Product4/2
  xy3/1 -> Add1/2, Add4/2, Add2/1
  Constant4/1 -> Product5/2
  Product6/1 -> Add/1
  Constant/1 -> Product6/1
  Constant1/1 -> Product1/1
  Product1/1 -> Add/2
  Add2/1 -> Product5/1
  Add5/1 -> Product6/2
  Add/1 -> p3y/1
  xy4/1 -> Add4/1
  xy1/1 -> Add2/2
  xy5/1 -> Add1/1
  Constant5/1 -> Product3/1
  Add1/1 -> Product3/2
  Product3/1 -> Add5/1
  Product7/1 -> Add9/1
  Add6/1 -> Product7/2
  Constant7/1 -> Product7/1
  vy5/1 -> Add6/1
  vy1/1 -> Add7/2
  vy4/1 -> Add8/1
  Add7/1 -> Product9/1
  Constant6/1 -> Product9/2
  vy3/1 -> Add7/1, Add8/2, Add6/2
  Add8/1 -> Product8/2
  Constant2/1 -> Product8/1
  Product9/1 -> Add9/3
  Product8/1 -> Add9/2

== system chap05/Subsystem16/Subsystem17/Subsystem2 ==
  xz3 : Inport
  xz1 : Inport  Port=2
  xz4 : Inport  Port=3
  xz5 : Inport  Port=4
  vz3 : Inport  Port=5
  vz1 : Inport  Port=6
  vz4 : Inport  Port=7
  vz5 : Inport  Port=8
  Add : Sum
  Add{1,4,6,8} (4 alike) : Sum  Inputs=-+
  Add2 : Sum  Inputs=+-
  Add5 : Sum  Inputs=+++
  Add7 : Sum  Inputs=+-
  Add9 : Sum  Inputs=+++
  Constant : Constant  Value=0.75
  Constant1 : Constant  Value=0.85
  Constant2 : Constant  Value=0.8
  Constant3 : Constant  Value=0.8
  Constant4 : Constant  Value=0.5
  Constant5 : Constant  Value=1.5
  Constant6 : Constant  Value=0.5
  Constant7 : Constant  Value=1.5
  Product{1,3..9} (8 alike) : Product
  p3z : Outport
  wires:
  Product8/1 -> Add9/2
  Product9/1 -> Add9/3
  Constant2/1 -> Product8/1
  Add8/1 -> Product8/2
  vz3/1 -> Add6/2, Add8/2, Add7/1
  Constant6/1 -> Product9/2
  Add7/1 -> Product9/1
  vz4/1 -> Add8/1
  vz1/1 -> Add7/2
  vz5/1 -> Add6/1
  Constant7/1 -> Product7/1
  Add6/1 -> Product7/2
  Product7/1 -> Add9/1
  Product3/1 -> Add5/1
  Add1/1 -> Product3/2
  Constant5/1 -> Product3/1
  xz5/1 -> Add1/1
  xz1/1 -> Add2/2
  xz4/1 -> Add4/1
  Add/1 -> p3z/1
  Add5/1 -> Product6/2
  Add2/1 -> Product5/1
  Product1/1 -> Add/2
  Constant1/1 -> Product1/1
  Constant/1 -> Product6/1
  Product6/1 -> Add/1
  Constant4/1 -> Product5/2
  xz3/1 -> Add2/1, Add4/2, Add1/2
  Add4/1 -> Product4/2
  Constant3/1 -> Product4/1
  Product5/1 -> Add5/3
  Product4/1 -> Add5/2
  Add9/1 -> Product1/2

== system chap05/Subsystem16/Subsystem17/Subsystem3 ==
  xyk : Inport
  xy : Inport  Port=2
  vyk : Inport  Port=3
  vy : Inport  Port=4
  Add : Sum
  Add4 : Sum  Inputs=-+
  Add8 : Sum  Inputs=-+
  Constant : Constant  Value=0.75
  Constant1 : Constant  Value=0.85
  Product1 : Product
  Product6 : Product
  ey : Outport
  wires:
  vyk/1 -> Add8/2
  vy/1 -> Add8/1
  xy/1 -> Add4/1
  Add/1 -> ey/1
  Add4/1 -> Product6/2
  Product1/1 -> Add/2
  Constant1/1 -> Product1/1
  Constant/1 -> Product6/1
  Product6/1 -> Add/1
  xyk/1 -> Add4/2
  Add8/1 -> Product1/2

== system chap05/Subsystem16/Subsystem17/Subsystem4 ==
  xzk : Inport
  xz : Inport  Port=2
  vzk : Inport  Port=3
  vz : Inport  Port=4
  Add : Sum
  Add4 : Sum  Inputs=-+
  Add8 : Sum  Inputs=-+
  Constant : Constant  Value=0.75
  Constant1 : Constant  Value=0.85
  Product1 : Product
  Product6 : Product
  ez : Outport
  wires:
  Add8/1 -> Product1/2
  xzk/1 -> Add4/2
  Product6/1 -> Add/1
  Constant/1 -> Product6/1
  Constant1/1 -> Product1/1
  Product1/1 -> Add/2
  Add4/1 -> Product6/2
  Add/1 -> ez/1
  xz/1 -> Add4/1
  vz/1 -> Add8/1
  vzk/1 -> Add8/2

== system chap05/Subsystem16/Subsystem17/Subsystem5 ==
  xxk : Inport
  xx : Inport  Port=2
  vxk : Inport  Port=3
  vx : Inport  Port=4
  Add : Sum
  Add4 : Sum  Inputs=-+
  Add8 : Sum  Inputs=-+
  Constant : Constant  Value=0.75
  Constant1 : Constant  Value=0.85
  Product1 : Product
  Product6 : Product
  ex : Outport
  wires:
  Add8/1 -> Product1/2
  xxk/1 -> Add4/2
  Product6/1 -> Add/1
  Constant/1 -> Product6/1
  Constant1/1 -> Product1/1
  Product1/1 -> Add/2
  Add4/1 -> Product6/2
  Add/1 -> ex/1
  xx/1 -> Add4/1
  vx/1 -> Add8/1
  vxk/1 -> Add8/2

== system chap05/Subsystem16/Subsystem17/Subsystem6 ==
  xx3 : Inport
  xx1 : Inport  Port=2
  xx4 : Inport  Port=3
  xx5 : Inport  Port=4
  vx3 : Inport  Port=5
  vx1 : Inport  Port=6
  vx4 : Inport  Port=7
  vx5 : Inport  Port=8
  Add : Sum
  Add{1,4,6,8} (4 alike) : Sum  Inputs=-+
  Add2 : Sum  Inputs=+-
  Add5 : Sum  Inputs=+++
  Add7 : Sum  Inputs=+-
  Add9 : Sum  Inputs=+++
  Constant : Constant  Value=0.75
  Constant1 : Constant  Value=0.85
  Constant2 : Constant  Value=0.8
  Constant3 : Constant  Value=0.8
  Constant4 : Constant  Value=0.5
  Constant5 : Constant  Value=1.5
  Constant6 : Constant  Value=0.5
  Constant7 : Constant  Value=1.5
  Product{1,3..9} (8 alike) : Product
  p3x : Outport
  wires:
  Product8/1 -> Add9/2
  Product9/1 -> Add9/3
  Constant2/1 -> Product8/1
  Add8/1 -> Product8/2
  vx3/1 -> Add6/2, Add8/2, Add7/1
  Constant6/1 -> Product9/2
  Add7/1 -> Product9/1
  vx4/1 -> Add8/1
  vx1/1 -> Add7/2
  vx5/1 -> Add6/1
  Constant7/1 -> Product7/1
  Add6/1 -> Product7/2
  Product7/1 -> Add9/1
  Product3/1 -> Add5/1
  Add1/1 -> Product3/2
  Constant5/1 -> Product3/1
  xx5/1 -> Add1/1
  xx1/1 -> Add2/2
  xx4/1 -> Add4/1
  Add/1 -> p3x/1
  Add5/1 -> Product6/2
  Add2/1 -> Product5/1
  Product1/1 -> Add/2
  Constant1/1 -> Product1/1
  Constant/1 -> Product6/1
  Product6/1 -> Add/1
  Constant4/1 -> Product5/2
  xx3/1 -> Add2/1, Add4/2, Add1/2
  Add4/1 -> Product4/2
  Constant3/1 -> Product4/1
  Product5/1 -> Add5/3
  Product4/1 -> Add5/2
  Add9/1 -> Product1/2

== system chap05/Subsystem16/Subsystem2/Subsystem1 ==
  xy2 : Inport
  xy1 : Inport  Port=2
  xy4 : Inport  Port=3
  xy6 : Inport  Port=4
  vy2 : Inport  Port=5
  vy1 : Inport  Port=6
  vy4 : Inport  Port=7
  vy6 : Inport  Port=8
  Add : Sum
  Add{1,4,6,8} (4 alike) : Sum  Inputs=-+
  Add2 : Sum  Inputs=+-
  Add5 : Sum  Inputs=+++
  Add7 : Sum  Inputs=+-
  Add9 : Sum  Inputs=+++
  Constant : Constant  Value=0.75
  Constant1 : Constant  Value=0.85
  Constant2 : Constant  Value=0.5
  Constant3 : Constant  Value=0.5
  Constant4 : Constant  Value=0.8
  Constant5 : Constant  Value=1.5
  Constant6 : Constant  Value=0.8
  Constant7 : Constant  Value=1.5
  Gain : Gain  Gain=-1
  Product{1,3..9} (8 alike) : Product
  p2y : Outport
  wires:
  Product8/1 -> Add9/2
  Product9/1 -> Add9/3
  Constant2/1 -> Product8/1
  Add8/1 -> Product8/2
  vy2/1 -> Add6/2, Add8/2, Add7/1
  Constant6/1 -> Product9/2
  Add7/1 -> Product9/1
  vy4/1 -> Add8/1
  vy1/1 -> Add7/2
  vy6/1 -> Add6/1
  Constant7/1 -> Product7/1
  Add6/1 -> Product7/2
  Product7/1 -> Add9/1
  Product3/1 -> Add5/1
  Add1/1 -> Product3/2
  Constant5/1 -> Product3/1
  xy6/1 -> Add1/1
  xy1/1 -> Add2/2
  xy4/1 -> Add4/1
  Add5/1 -> Product6/2
  Add2/1 -> Product5/1
  Product1/1 -> Add/2
  Constant1/1 -> Product1/1
  Constant/1 -> Product6/1
  Product6/1 -> Add/1
  Constant4/1 -> Product5/2
  xy2/1 -> Add2/1, Add4/2, Add1/2
  Add4/1 -> Product4/2
  Constant3/1 -> Product4/1
  Product5/1 -> Add5/3
  Product4/1 -> Add5/2
  Add9/1 -> Product1/2
  Gain/1 -> p2y/1
  Add/1 -> Gain/1

== system chap05/Subsystem16/Subsystem2/Subsystem10 ==
  utx : Inport
  uty : Inport  Port=2
  utz : Inport  Port=3
  Add : Sum
  Constant3 : Constant
  Constant4 : Constant  Value=0
  Data Store Memory : DataStoreMemory  DataStoreName=utkz2  ReadBeforeWriteMsg=warning  WriteAfterWriteMsg=warning  WriteAfterReadMsg=warning  ShowAdditionalParam=off
  Data Store Memory1 : DataStoreMemory  DataStoreName=utky2  ReadBeforeWriteMsg=warning  WriteAfterWriteMsg=warning  WriteAfterReadMsg=warning  ShowAdditionalParam=off
  Data Store Memory2 : DataStoreMemory  DataStoreName=utkx2  ReadBeforeWriteMsg=warning  WriteAfterWriteMsg=warning  WriteAfterReadMsg=warning  ShowAdditionalParam=off
  Data Store Memory3 : DataStoreMemory  DataStoreName=uc2  ReadBeforeWriteMsg=warning  WriteAfterWriteMsg=warning  WriteAfterReadMsg=warning  ShowAdditionalParam=off
  Data Store Read : DataStoreRead  DataStoreName=uc2  IndexOptions=Index vector (dialog)  Indices=1  OutputSizes=1
  Data Store Read1 : DataStoreRead  DataStoreName=utkx2  IndexOptions=Index vector (dialog)  Indices=1  OutputSizes=1
  Data Store Read2 : DataStoreRead  DataStoreName=utky2  IndexOptions=Index vector (dialog)  Indices=1  OutputSizes=1
  Data Store Read3 : DataStoreRead  DataStoreName=utkz2  IndexOptions=Index vector (dialog)  Indices=1  OutputSizes=1
  Data Store Write : DataStoreWrite  DataStoreName=uc2  IndexOptions=Index vector (dialog)  Indices=1  OutputSizes=1
  Data Store Write1 : DataStoreWrite  DataStoreName=utkx2  IndexOptions=Index vector (dialog)  Indices=1  OutputSizes=1
  Data Store Write2 : DataStoreWrite  DataStoreName=utky2  IndexOptions=Index vector (dialog)  Indices=1  OutputSizes=1
  Data Store Write3 : DataStoreWrite  DataStoreName=utkz2  IndexOptions=Index vector (dialog)  Indices=1  OutputSizes=1
  Demux : Demux  Outputs=3
  Display : Display
  MATLAB Function : MATLAB Function  TreatAsAtomicUnit=on
  Mux1 : Mux  Inputs=3
  Mux2 : Mux  Inputs=3
  Switch : Switch  Threshold=0.1
  Switch2 : Switch  Threshold=0.1
  ux : Outport
  uy : Outport  Port=2
  uz : Outport  Port=3
  wires:
  Mux2/1 -> [utk], MATLAB Function/2(utk)
  Mux1/1 -> [ut], MATLAB Function/1(u)
  Switch/1 -> Demux/1
  Data Store Read1/1 -> Mux2/1
  Data Store Read3/1 -> Mux2/3
  Data Store Read2/1 -> Mux2/2
  Demux/3 -> Data Store Write3/1, uz/1
  Demux/1 -> Data Store Write1/1, ux/1
  Add/1 -> Data Store Write/1, Display/1
  Data Store Read/1 -> Add/2
  Switch2/1 -> Add/1  "e1"
  Constant3/1 -> Switch2/1
  Constant4/1 -> Switch2/3
  MATLAB Function/1(nrom) -> Switch2/2, Switch/2
  utx/1 -> Mux1/1
  uty/1 -> Mux1/2
  utz/1 -> Mux1/3
  Demux/2 -> Data Store Write2/1, uy/1
  [ut] -> Switch/1
  [utk] -> Switch/3

== system chap05/Subsystem16/Subsystem2/Subsystem11 ==
  vz2 : Inport
  utz : Inport  Port=2
  gain : Inport  Port=3
  switch : Inport  Port=4
  Add1 : Sum  Inputs=--+
  Constant1 : Constant  Value=0.08
  Constant2 : Constant  Value=10
  Product : Product
  Product1 : Product
  Product2 : Product
  Subsystem : Subsystem
  Subtract : Sum  Inputs=+-
  Switch1 : Switch  Criteria=u2 > Threshold  Threshold=1
  Tanh : Trigonometry  Operator=tanh
  uz : Outport
  Sz : Outport  Port=2
  wires:
  Add1/1 -> Switch1/1
  utz/1 -> [A], Subsystem/2(zt3)
  Product/1 -> Add1/2
  vz2/1 -> Subtract/1
  Product2/1 -> Tanh/1
  Tanh/1 -> Product/1
  gain/1 -> Product/2
  [A] -> Add1/3
  Constant2/1 -> Product2/2
  Product1/1 -> Add1/1
  Subtract/1 -> Sz/1, Product1/2, Product2/1
  Subsystem/1(Out1) -> Subtract/2
  switch/1 -> [switch], Subsystem/1(switch)
  [A] -> Switch1/3
  [switch] -> Switch1/2
  Switch1/1 -> uz/1
  Constant1/1 -> Product1/1

== system chap05/Subsystem16/Subsystem2/Subsystem2 ==
  xz2 : Inport
  xz1 : Inport  Port=2
  xz4 : Inport  Port=3
  xz6 : Inport  Port=4
  vz2 : Inport  Port=5
  vz1 : Inport  Port=6
  vz4 : Inport  Port=7
  vz6 : Inport  Port=8
  Add : Sum
  Add{1,4,6,8} (4 alike) : Sum  Inputs=-+
  Add2 : Sum  Inputs=+-
  Add5 : Sum  Inputs=+++
  Add7 : Sum  Inputs=+-
  Add9 : Sum  Inputs=+++
  Constant : Constant  Value=0.75
  Constant1 : Constant  Value=0.85
  Constant2 : Constant  Value=0.5
  Constant3 : Constant  Value=0.5
  Constant4 : Constant  Value=0.8
  Constant5 : Constant  Value=1.5
  Constant6 : Constant  Value=0.8
  Constant7 : Constant  Value=1.5
  Gain : Gain  Gain=-1
  Product{1,3..9} (8 alike) : Product
  p2z : Outport
  wires:
  Add9/1 -> Product1/2
  Product4/1 -> Add5/2
  Product5/1 -> Add5/3
  Constant3/1 -> Product4/1
  Add4/1 -> Product4/2
  xz2/1 -> Add1/2, Add4/2, Add2/1
  Constant4/1 -> Product5/2
  Product6/1 -> Add/1
  Constant/1 -> Product6/1
  Constant1/1 -> Product1/1
  Product1/1 -> Add/2
  Add2/1 -> Product5/1
  Add5/1 -> Product6/2
  xz4/1 -> Add4/1
  xz1/1 -> Add2/2
  xz6/1 -> Add1/1
  Constant5/1 -> Product3/1
  Add1/1 -> Product3/2
  Product3/1 -> Add5/1
  Product7/1 -> Add9/1
  Add6/1 -> Product7/2
  Constant7/1 -> Product7/1
  vz6/1 -> Add6/1
  vz1/1 -> Add7/2
  vz4/1 -> Add8/1
  Add7/1 -> Product9/1
  Constant6/1 -> Product9/2
  vz2/1 -> Add7/1, Add8/2, Add6/2
  Add8/1 -> Product8/2
  Constant2/1 -> Product8/1
  Product9/1 -> Add9/3
  Product8/1 -> Add9/2
  Gain/1 -> p2z/1
  Add/1 -> Gain/1

== system chap05/Subsystem16/Subsystem2/Subsystem3 ==
  utx : Inport
  vx : Inport  Port=2
  vy : Inport  Port=3
  vz : Inport  Port=4
  uty : Inport  Port=5
  ux : Inport  Port=6
  uy : Inport  Port=7
  uz : Inport  Port=8
  utz : Inport  Port=9
  switch : Inport  Port=10
  Add3 : Sum  Inputs=-+
  Add4 : Sum  Inputs=-+
  Add5 : Sum  Inputs=-+
  Demux : Demux  Outputs=3
  Demux1 : Demux  Outputs=3
  Discrete-Time Integrator1 : DiscreteIntegrator  SampleTime=-1  ICPrevOutput=DiscIntNeverNeededParam  ICPrevScaledInput=DiscIntNeverNeededParam
  Discrete-Time Integrator2 : DiscreteIntegrator  SampleTime=-1  ICPrevOutput=DiscIntNeverNeededParam  ICPrevScaledInput=DiscIntNeverNeededParam
  Discrete-Time Integrator8 : DiscreteIntegrator  SampleTime=-1  ICPrevOutput=DiscIntNeverNeededParam  ICPrevScaledInput=DiscIntNeverNeededParam
  MATLAB Function : MATLAB Function  TreatAsAtomicUnit=on
  MATLAB Function1 : MATLAB Function  TreatAsAtomicUnit=on
  MATLAB Function2 : MATLAB Function  TreatAsAtomicUnit=on
  Mux : Mux  Inputs=3
  Mux1 : Mux  Inputs=3
  Subsystem : Subsystem
  Subsystem1 : Subsystem
  Subsystem2 : Subsystem
      settings: PortSchema="{\"entries\":[{\"content\":{\"sides\":[{\"content\":{\"connectorIds\":[\"In1\"]},\"type\":\"ConnectorPlacement.EquallySpacedRectSide\",\"uuid\":\"fc08b57d-5108-4bb3-894e-d1527c9ee9b9\"},{\"content\":{\"connectorIds\":[\"Out1\",\"Out2\",\"Out3\",\"Out4\"],\"side\":\"RIGHT\"},\"type\":\"ConnectorPlacement.EquallySpacedRectSide\",\"uuid\":\"5f28f464-9d6d-4ee7-848e-113b4b51ead6\"},{\"content\":{\"connectorIds\":[],\"side\":\"TOP\"},\"type\":\"ConnectorPlacement.EquallySpacedRectSide\",\"uuid\":\"5cca314e-822b-43eb-ac4d-78622e8ed582\"},{\"content\":{\"connectorIds\":[\"In2\"],\"side\":\"BOTTOM\"},\"type\":\"ConnectorPlacement.EquallySpacedRectSide\",\"uuid\":\"aa07b2d0-4f6e-4d8e-96de-14c35ee3da88\"}]},\"type\":\"ConnectorPlacement.EquallySpacedConnector\",\"uuid\":\"246d6f2c-2f9e-403c-b810-eff9b0fc0735\"}],\"packageUris\":[\"http://schema.mathworks.com/mf0/Connector/R2020b\"],\"version\":\"1.0\"}"
  Subsystem3 : Subsystem
  Subtract1 : Sum  Inputs=++++
  Subtract2 : Sum  Inputs=+-
  Subtract3 : Sum  Inputs=+-
  Subtract4 : Sum  Inputs=+-
  Switch1 : Switch  Criteria=u2 > Threshold  Threshold=1
  Switch2 : Switch  Criteria=u2 > Threshold  Threshold=1
  Switch3 : Switch  Criteria=u2 > Threshold  Threshold=1
  udtx : Outport
  udty : Outport  Port=2
  udtz : Outport  Port=3
  wires:
  Subsystem3/1(Out1) -> Subtract1/2
  Subsystem2/2(k2) -> Subsystem3/2(k2)
  Subsystem1/1(Out1) -> Subtract1/1
  Subsystem2/1(k1) -> Subsystem1/2(k1)
  Subtract4/1 -> MATLAB Function2/1(u)
  Subtract3/1 -> MATLAB Function1/1(u)
  Subtract2/1 -> MATLAB Function/1(u)
  Demux/3 -> Discrete-Time Integrator8/1
  Demux/1 -> Discrete-Time Integrator2/1
  Demux/2 -> Discrete-Time Integrator1/1
  Discrete-Time Integrator2/1 -> Subtract2/1
  Discrete-Time Integrator1/1 -> Subtract3/1
  Discrete-Time Integrator8/1 -> Subtract4/1
  Mux1/1 -> Subtract1/4
  ux/1 -> Mux1/1
  uy/1 -> Mux1/2
  uz/1 -> Mux1/3
  vx/1 -> Subtract2/2
  Subsystem2/4(k4) -> Subsystem/3(k4)
  Subsystem/1(z2) -> Subtract1/3, Demux1/1  "od2"
  Subsystem2/3(k3) -> Subsystem/2(k3)
  Subtract1/1 -> Demux/1
  Mux/1 -> Subsystem1/1(e1), Subsystem3/1(e1), Subsystem2/1(e1), Subsystem/1(e1)
  utx/1 -> Switch1/3, Add3/2
  uty/1 -> Switch2/3, Add5/2
  utz/1 -> Switch3/3, Add4/2
  vy/1 -> Subtract3/2
  vz/1 -> Subtract4/2
  MATLAB Function/1(y) -> Mux/1
  MATLAB Function1/1(y) -> Mux/2
  MATLAB Function2/1(y) -> Mux/3
  switch/1 -> [switch], Switch3/2, Switch1/2, Switch2/2
  [switch] -> Subsystem2/2(switch)
  Add3/1 -> Switch1/1
  Add5/1 -> Switch2/1
  Add4/1 -> Switch3/1
  Switch1/1 -> udtx/1
  Switch2/1 -> udty/1
  Switch3/1 -> udtz/1
  Demux1/1 -> Add3/1
  Demux1/2 -> Add5/1
  Demux1/3 -> Add4/1

== system chap05/Subsystem16/Subsystem2/Subsystem4 ==
  vx2 : Inport
  utx : Inport  Port=2
  gain : Inport  Port=3
  switch : Inport  Port=4
  Add1 : Sum  Inputs=--+
  Constant1 : Constant  Value=0.08
  Constant2 : Constant  Value=10
  Product : Product
  Product1 : Product
  Product2 : Product
  Subsystem : Subsystem
  Subtract : Sum  Inputs=+-
  Switch1 : Switch  Criteria=u2 > Threshold  Threshold=1
  Tanh : Trigonometry  Operator=tanh
  ux : Outport
  Sx : Outport  Port=2
  wires:
  Add1/1 -> Switch1/1
  utx/1 -> [A], Subsystem/2(zt3)
  Product/1 -> Add1/2
  vx2/1 -> Subtract/1
  Product2/1 -> Tanh/1
  Tanh/1 -> Product/1
  gain/1 -> Product/2
  [A] -> Add1/3
  Constant2/1 -> Product2/2
  Product1/1 -> Add1/1
  Constant1/1 -> Product1/1
  Subtract/1 -> Sx/1, Product1/2, Product2/1
  switch/1 -> [switch], Subsystem/1(switch)
  [A] -> Switch1/3
  [switch] -> Switch1/2
  Switch1/1 -> ux/1
  Subsystem/1(Out1) -> Subtract/2

== system chap05/Subsystem16/Subsystem2/Subsystem6 ==
  xx2 : Inport
  xx1 : Inport  Port=2
  xx4 : Inport  Port=3
  xx6 : Inport  Port=4
  vx2 : Inport  Port=5
  vx1 : Inport  Port=6
  vx4 : Inport  Port=7
  vx6 : Inport  Port=8
  Add : Sum
  Add{1,4,6,8} (4 alike) : Sum  Inputs=-+
  Add2 : Sum  Inputs=+-
  Add5 : Sum  Inputs=+++
  Add7 : Sum  Inputs=+-
  Add9 : Sum  Inputs=+++
  Constant : Constant  Value=0.75
  Constant1 : Constant  Value=0.85
  Constant2 : Constant  Value=0.5
  Constant3 : Constant  Value=0.5
  Constant4 : Constant  Value=0.8
  Constant5 : Constant  Value=1.5
  Constant6 : Constant  Value=0.8
  Constant7 : Constant  Value=1.5
  Gain : Gain  Gain=-1
  Product{1,3..9} (8 alike) : Product
  p2x : Outport
  wires:
  Add9/1 -> Product1/2
  Product4/1 -> Add5/2
  Product5/1 -> Add5/3
  Constant3/1 -> Product4/1
  Add4/1 -> Product4/2
  xx2/1 -> Add1/2, Add4/2, Add2/1
  Constant4/1 -> Product5/2
  Product6/1 -> Add/1
  Constant/1 -> Product6/1
  Constant1/1 -> Product1/1
  Product1/1 -> Add/2
  Add2/1 -> Product5/1
  Add5/1 -> Product6/2
  xx4/1 -> Add4/1
  xx1/1 -> Add2/2
  xx6/1 -> Add1/1
  Constant5/1 -> Product3/1
  Add1/1 -> Product3/2
  Product3/1 -> Add5/1
  Product7/1 -> Add9/1
  Add6/1 -> Product7/2
  Constant7/1 -> Product7/1
  vx6/1 -> Add6/1
  vx1/1 -> Add7/2
  vx4/1 -> Add8/1
  Add7/1 -> Product9/1
  Constant6/1 -> Product9/2
  vx2/1 -> Add7/1, Add8/2, Add6/2
  Add8/1 -> Product8/2
  Constant2/1 -> Product8/1
  Product9/1 -> Add9/3
  Product8/1 -> Add9/2
  Gain/1 -> p2x/1
  Add/1 -> Gain/1
